simulink model "MainorMatlab"  (R2023a)
settings: Solver=VariableStepAuto  StartTime=0.0  StopTime=10.0  RelTol=1e-3
settings Model: Creator=Hp  LastModifiedBy=Hp

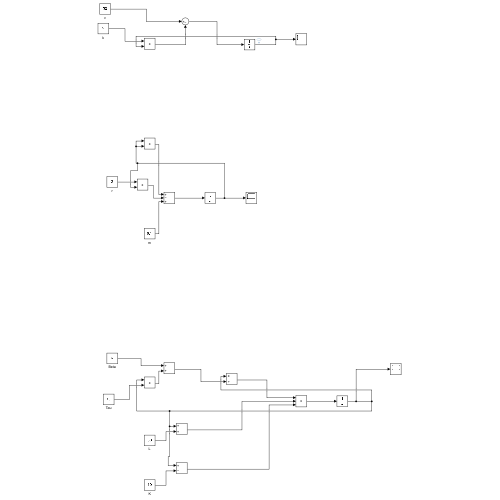
[thumbnail: Simulink's stored preview of the top-level diagram]
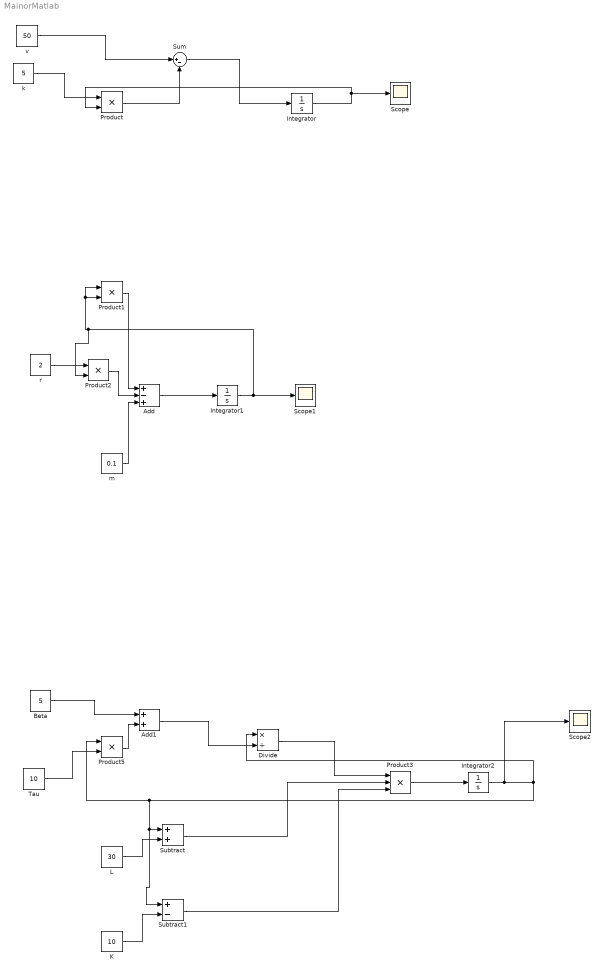
== system MainorMatlab ==
  Add : Sum  Inputs=+-+
  Add1 : Sum
  Beta : Constant  Value=5
  Divide : Product  Inputs=*/
  Integrator : Integrator  InitialCondition=1000
  Integrator1 : Integrator
  Integrator2 : Integrator  InitialCondition=25
  K : Constant  Value=10
  L : Constant  Value=30
  Product{,1..2,5} (4 alike) : Product
  Product3 : Product  Inputs=3
  Scope : Scope
  Scope1 : Scope
  Scope2 : Scope
  Subtract : Sum
  Subtract1 : Sum  Inputs=+-
  Sum : Sum  Inputs=|+-
  Tau : Constant  Value=10
  k : Constant  Value=5
  m : Constant  Value=0.1
  r : Constant  Value=2
  v : Constant  Value=50
  wires:
  k/1 -> Product/1
  Integrator/1 -> Product/2, Scope/1
  Product/1 -> Sum/2
  v/1 -> Sum/1
  Sum/1 -> Integrator/1
  m/1 -> Add/3
  Add/1 -> Integrator1/1
  r/1 -> Product2/1
  Product1/1 -> Add/1
  Product2/1 -> Add/2
  Integrator1/1 -> Product2/2, Product1/1, Product1/2, Scope1/1
  L/1 -> Subtract/2
  K/1 -> Subtract1/2
  Tau/1 -> Product5/2
  Product5/1 -> Add1/2
  Beta/1 -> Add1/1
  Product3/1 -> Integrator2/1
  Integrator2/1 -> Scope2/1, Divide/1, Product5/1, Subtract1/1, Subtract/1
  Add1/1 -> Divide/2
  Divide/1 -> Product3/1
  Subtract/1 -> Product3/2
  Subtract1/1 -> Product3/3
